simulink model "prMotor"  (R2021a)
settings: Solver=ode3  StartTime=0.0  StopTime=2  FixedStep=0.000125  RelTol=1e-3  EnableMultiTasking=on
values from neighbouring files (symbols this model uses):
  DELTA_EMF = 14    [prMotor_init.m]
  DELTA_THETA = 29    [prMotor_init.m]
  DT_GAIN = 102    [prMotor_init.m]
  DT_IREF_LIM = 205    [prMotor_init.m]
  DT_SET_H = 10    [prMotor_init.m]
  DT_SET_L = -10    [prMotor_init.m]
  DT_VALUE = 2    [prMotor_init.m]
  DUTY = 2048    [prMotor_init.m]
  DUTY_50 = 1024    [prMotor_init.m]
  EMF_GAIN = 759    [prMotor_init.m]
  ID_GAIN = 350    [prMotor_init.m]
  ID_LIM = 205    [prMotor_init.m]
  ID_RPM = 1800    [prMotor_init.m]
  IREF_FLT_A1 = -446    [prMotor_init.m]
  IREF_FLT_B0 = 289    [prMotor_init.m]
  IREF_FLT_B1 = 289    [prMotor_init.m]
  Ki = 0.048828125    [prMotor_init.m]
  mp_emf = [0	3	5	8	10	13	15	18	21	23	26	28	31	33	36	39	41	44	46	49	51	54	56	59	62	64	67	69	72	74	77	79	82	84	87	89	92	94	97	99	102	104	107	109	112	114	117	119	122	124	127	129	132	134	136	139	141	144	146	149	151	153	156	158	161	163	165	168	170	172	175	177	179	182	184	186	189	191	193	195	198	200	202	204	207	209	211	213	216	218	220	222	224	227	229	231	233	235	237	239	242	244	246	248	250	252	254	256	258	260	262 ...(+4035 chars)    [prMotor_init.m]
  mp_sin = [0	6	13	19	25	31	38	44	50	57	63	69	75	82	88	94	100	107	113	119	125	132	138	144	150	156	163	169	175	181	187	194	200	206	212	218	224	230	237	243	249	255	261	267	273	279	285	291	297	303	309	315	321	327	333	339	345	351	357	363	369	374	380	386	392	398	403	409	415	421	426	432	438	443	449	455	460	466	472	477	483	488	494	499	505	510	516	521	526	532	537	543	548	553	558	564	569	574	579	584	590	595	600	605	6 ...(+4281 chars)    [prMotor_init.m]
  mp_theta = [0	1	2	3	4	5	6	7	8	9	10	11	12	13	14	15	16	17	18	19	20	21	22	23	24	25	26	27	28	29	30	31	32	33	34	35	36	37	38	39	40	41	42	43	44	45	46	47	48	49	50	51	52	53	54	55	56	57	58	59	60	61	62	63	64	65	66	67	68	69	70	71	72	73	74	75	76	77	78	79	80	81	82	83	84	85	86	87	88	89	90	91	92	93	94	95	96	97	98	99	100	101	102	103	104	105	106	107	108	109	110	111	112	113	114	115	116	117	118	119	120	121	122	123	124	125	126	1 ...(+3610 chars)    [prMotor_init.m]
  PI_A1 = -1024    [prMotor_init.m]
  PI_B0 = 292    [prMotor_init.m]
  PI_B1 = -279    [prMotor_init.m]
  RPM_GAIN = 15000    [prMotor_init.m]
  RPM_LIM = 3000    [prMotor_init.m]
  RPM_LPF_A1 = -984    [prMotor_init.m]
  RPM_LPF_B0 = 20    [prMotor_init.m]
  RPM_LPF_B1 = 20    [prMotor_init.m]
  T_smp = 0.000125    [prMotor_init.m]
  THETA_ADV_LIM = 85    [prMotor_init.m]
libraries: simulink x1
(part 1 of 2)
settings Model: ModifiedByFormat=GAIO  Creator=GAIO  LastModifiedBy=GAIO
settings SolverCC: AlgebraicLoopSolver=TrustRegion
settings DataIOCC: LimitDataPoints=on  SaveFormat=Array  SignalLoggingSaveFormat=ModelDataLogs  SaveOutput=off  SaveTime=off  ReturnWorkspaceOutputs=off
settings OptimizationCC: ExpressionDepthLimit=2147483647  LifeSpan=1  EfficientTunableParamExpr=on
settings DebuggingCC: UnderspecifiedInitializationDetection=Classic  MergeDetectMultiDrivingBlocksExec=none  SolverPrmCheckMsg=warning  MultiTaskDSMMsg=warning  MultiTaskCondExecSysMsg=none  FcnCallInpInsideContextMsg=warning  StateNameClashWarn=warning  SFUnexpectedBacktrackingDiag=warning  SFNoUnconditionalDefaultTransitionDiag=warning  SFExecutionAtInitializationDiag=none  SFMachineParentedDataDiag=warning  ArithmeticOperatorsInVariantConditions=warning
settings HardwareCC: ProdBitPerPointer=32  ProdBitPerSizeT=32  ProdBitPerPtrDiffT=32  ProdLargestAtomicFloat=None  ProdIntDivRoundTo=Undefined  ProdEndianess=Unspecified  ProdWordSize=32  ProdHWDeviceType=32-bit Generic
settings ModelReferenceCC: PropagateSignalLabelsOutOfModel=off
settings SFSimCC: SimUseLocalCustomCode=off  MATLABDynamicMemAlloc=off  CustomCodeUndefinedFunction=UseInterfaceOnly
settings RTWCC: SystemTargetFile=ert.tlc  TemplateMakefile=ert_default_tmf  RTWUseLocalCustomCode=off
settings CodeAppCC: IgnoreCustomStorageClasses=off  StateflowObjectComments=on
settings ERTTargetCC: MultiwordLength=2048  GenerateSampleERTMain=on  SupportContinuousTime=on  ERTCustomFileTemplate=example_file_process.tlc  ConvertIfToSwitch=off  SuppressUnreachableDefaultCases=off
settings ConfigComp: CovMetricSettings=dcmtrzoibsw  CovSaveCumulativeToWorkspaceVar=on  CovSaveSingleToWorkspaceVar=on  CovSFcnEnable=off  DVMaxProcessTime=7200  DVTestSuiteOptimization=CombinedObjectives (Nonlinear Extended)  DVDetectOutOfBounds=on  DVSaveReport=on

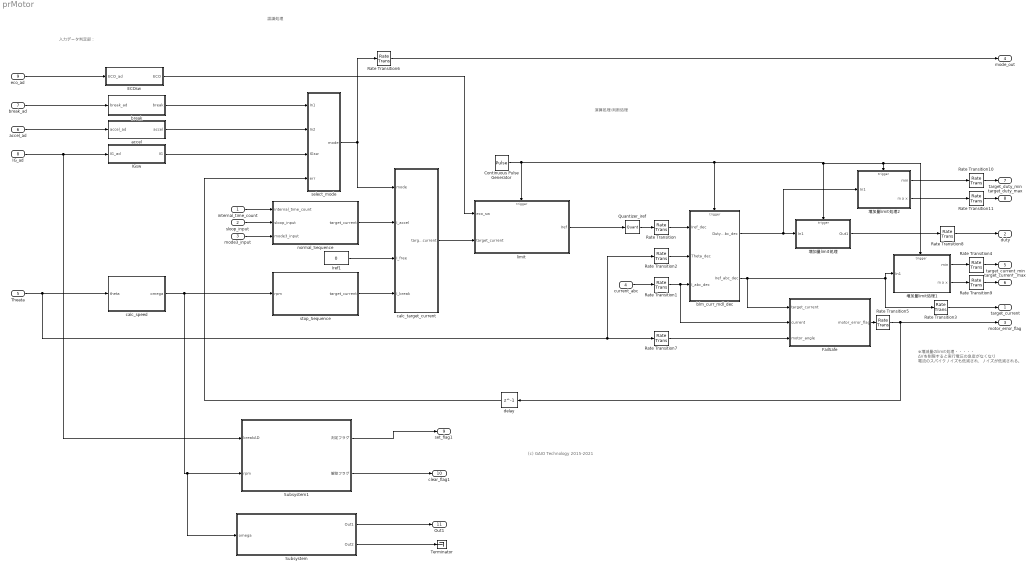
== system prMotor ==
  note: (c) GAIO Technology 2015-2021
  note: 認識処理
  note: 演算処理/判断処理
  note: 入力データ判定部：
  note: ※増減量のlimit処理・・・・・
      | ΔVを制限すると実行電圧の急変がなくなり
      | 電流のスパイクノイズも低減され、ノイズが低減される。
  internal_time_count : Inport  OutDataTypeStr=double  PortDimensions=1  SampleTime=[0.000125,0]
  sloop_input : Inport  Port=2  OutDataTypeStr=double  PortDimensions=1  SampleTime=[0.000125,0]
  mode3_input : Inport  Port=3  OutDataTypeStr=double  PortDimensions=1  SampleTime=[0.000125,0]
  current_abc : Inport  Port=4  OutDataTypeStr=double  PortDimensions=3  SampleTime=[0.000125,0]
  Theata : Inport  Port=5  OutDataTypeStr=double  PortDimensions=1  SampleTime=[0.000125,0]
  accel_ad : Inport  Port=6  SampleTime=[0.000125,0]
  break_ad : Inport  Port=7  SampleTime=[0.000125,0]
  IG_ad : Inport  Port=8  SampleTime=[0.000125,0]
  eco_ad : Inport  Port=9  SampleTime=[0.000125,0]
  Continuous Pulse Generator : DiscretePulseGenerator  PulseType=Time based  Period=T_smp*2  PulseWidth=50
  ECOsw : Subsystem
  FailSafe : Subsystem
  IGsw : Subsystem
  Iref1 : Constant  Value=0
  Quantizer_iref : Quantizer  QuantizationInterval=1
  Rate Transition{,1..4,6..11} (11 alike) : RateTransition
  Rate Transition5 : RateTransition  OutPortSampleTimeOpt=Inherit
  Subsystem : Subsystem
  Subsystem1 : Subsystem
  Terminator : Terminator
  accel : Subsystem
  blm_curr_mdl_dec : Subsystem
  break : Subsystem
  calc_speed : Subsystem
  calc_target_current : Subsystem
  delay : Delay  DelayLength=1  InitialCondition=0
  limit : Subsystem  TreatAsAtomicUnit=on
  normal_Sequence : Subsystem
  select_mode : Subsystem
  stop_Sequence : Subsystem
  増加量limit処理 : Subsystem
  増加量limit処理1 : Subsystem
  増加量limit処理2 : Subsystem
  target_current : Outport  OutDataTypeStr=double  PortDimensions=3  SampleTime=[0.000125,0]
  duty : Outport  Port=2  OutDataTypeStr=double  PortDimensions=3  SampleTime=[0.000125,0]
  motor_error_flag : Outport  Port=3  OutDataTypeStr=boolean  PortDimensions=1  SampleTime=[0.000125,0]
  mode_out : Outport  Port=4  OutDataTypeStr=double  PortDimensions=1  SampleTime=[0.000125,0]
  target_current_min : Outport  Port=5  OutDataTypeStr=double  PortDimensions=3  SampleTime=[0.000125,0]
  target_current＿max : Outport  Port=6  OutDataTypeStr=double  PortDimensions=3  SampleTime=[0.000125,0]
  target_duty_min : Outport  Port=7  OutDataTypeStr=double  PortDimensions=3  SampleTime=[0.000125,0]
  target_duty_max : Outport  Port=8  OutDataTypeStr=double  PortDimensions=3  SampleTime=[0.000125,0]
  set_flag1 : Outport  Port=9  OutDataTypeStr=boolean  PortDimensions=1  SampleTime=[0.000125,0]
  clear_flag1 : Outport  Port=10  OutDataTypeStr=boolean  PortDimensions=1  SampleTime=[0.000125,0]
  Out1 : Outport  Port=11
  wires:
  Rate Transition2/1 -> blm_curr_mdl_dec/2(Theta_dec)
  Rate Transition1/1 -> FailSafe/2(current), blm_curr_mdl_dec/3(I_abc_dec)
  Continuous Pulse Generator/1 -> 増加量limit処理2/Trigger, 増加量limit処理1/Trigger, 増加量limit処理/Trigger, blm_curr_mdl_dec/Trigger, limit/Trigger
  Rate Transition/1 -> blm_curr_mdl_dec/1(Iref_dec)
  current_abc/1 -> Rate Transition1/1
  Quantizer_iref/1 -> Rate Transition/1
  blm_curr_mdl_dec/2(Iref_abc_dec) -> Rate Transition3/1, 増加量limit処理1/1(In1), FailSafe/1(target_current)
  blm_curr_mdl_dec/1(Duty_abc_dec) -> 増加量limit処理2/1(In1), 増加量limit処理/1(In1)
  limit/1(Iref) -> Quantizer_iref/1
  FailSafe/1(motor_error_flag) -> Rate Transition5/1
  Rate Transition5/1 -> motor_error_flag/1, delay/1
  accel_ad/1 -> accel/1(accel_ad)
  break_ad/1 -> break/1(break_ad)
  Rate Transition6/1 -> mode_out/1
  break/1(break) -> select_mode/1(In1)
  accel/1(accel) -> select_mode/2(In2)
  select_mode/1(mode) -> Rate Transition6/1, calc_target_current/1(mode)
  internal_time_count/1 -> normal_Sequence/1(internal_time_count)
  mode3_input/1 -> normal_Sequence/3(mode3_input)
  sloop_input/1 -> normal_Sequence/2(sloop_input)
  normal_Sequence/1(target_current) -> calc_target_current/2(I_accel)
  Iref1/1 -> calc_target_current/3(I_free)
  stop_Sequence/1(target_current) -> calc_target_current/4(I_break)
  Theata/1 -> Rate Transition7/1, Rate Transition2/1, calc_speed/1(theta)
  calc_speed/1(omega) -> Subsystem/1(omega), Subsystem1/2(rpm), stop_Sequence/1(rpm)
  IG_ad/1 -> Subsystem1/1(breakAD), IGsw/1(IG_ad)
  IGsw/1(IG) -> select_mode/3(IGsw)
  Rate Transition7/1 -> FailSafe/3(motor_angle)
  calc_target_current/1(target_current) -> limit/2(target_current)
  eco_ad/1 -> ECOsw/1(ECO_ad)
  ECOsw/1(ECO) -> limit/1(eco_sw)
  delay/1 -> select_mode/4(err)
  増加量limit処理/1(Out1) -> Rate Transition8/1
  増加量limit処理1/1(min) -> Rate Transition4/1
  増加量limit処理1/2(ｍａｘ) -> Rate Transition9/1
  Rate Transition8/1 -> duty/1
  Rate Transition3/1 -> target_current/1
  Rate Transition4/1 -> target_current_min/1
  Rate Transition9/1 -> target_current＿max/1
  Rate Transition11/1 -> target_duty_max/1
  Rate Transition10/1 -> target_duty_min/1
  増加量limit処理2/2(ｍａｘ) -> Rate Transition11/1
  増加量limit処理2/1(min) -> Rate Transition10/1
  Subsystem1/1(判定フラグ) -> set_flag1/1
  Subsystem1/2("解除フラグ　") -> clear_flag1/1
  Subsystem/1(Out1) -> Out1/1
  Subsystem/2(Out2) -> Terminator/1

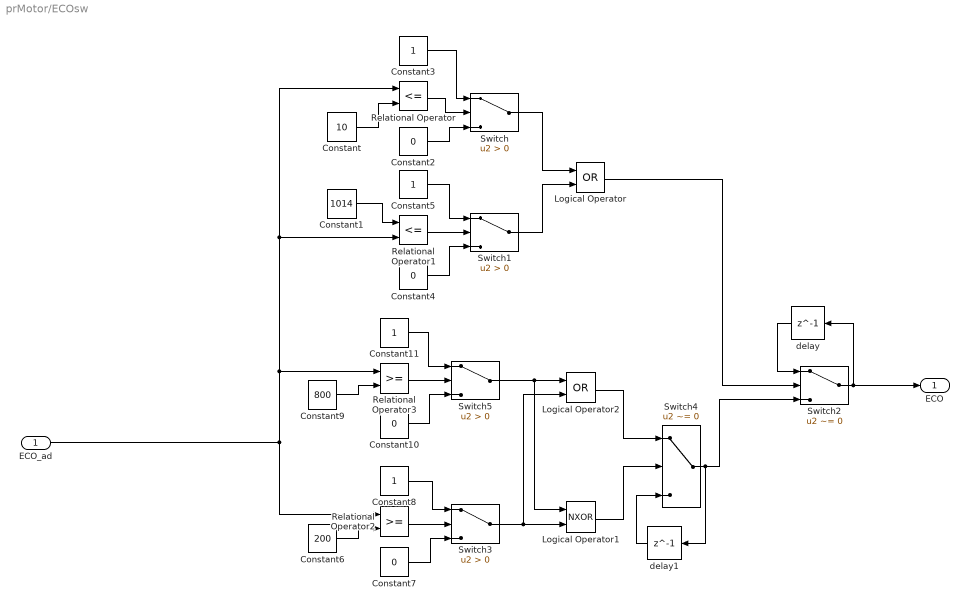
== system prMotor/ECOsw ==
  ECO_ad : Inport
  Constant : Constant  Value=10
  Constant1 : Constant  Value=1014
  Constant{2,4,7,10} (4 alike) : Constant  Value=0
  Constant{3,5,8,11} (4 alike) : Constant
  Constant6 : Constant  Value=200
  Constant9 : Constant  Value=800
  Logical Operator : Logic  Operator=OR  AllPortsSameDT=off  OutDataTypeStr=boolean
  Logical Operator1 : Logic  Operator=NXOR  AllPortsSameDT=off  OutDataTypeStr=boolean
  Logical Operator2 : Logic  Operator=OR  AllPortsSameDT=off  OutDataTypeStr=boolean
  Relational Operator : RelationalOperator  Operator=<=  OutDataTypeStr=boolean  RndMeth=Nearest
  Relational Operator1 : RelationalOperator  Operator=<=  OutDataTypeStr=boolean  RndMeth=Nearest
  Relational Operator2 : RelationalOperator  OutDataTypeStr=boolean  RndMeth=Nearest
  Relational Operator3 : RelationalOperator  OutDataTypeStr=boolean  RndMeth=Nearest
  Switch{,1,3,5} (4 alike) : Switch  Criteria=u2 > Threshold
  Switch2 : Switch  Criteria=u2 ~= 0
  Switch4 : Switch  Criteria=u2 ~= 0
  delay : Delay  DelayLength=1  InitialCondition=0
  delay1 : Delay  DelayLength=1  InitialCondition=0
  ECO : Outport
  wires:
  Logical Operator2/1 -> Switch4/1
  Logical Operator1/1 -> Switch4/2
  ECO_ad/1 -> Relational Operator2/1, Relational Operator3/1, Relational Operator/1, Relational Operator1/2
  Constant10/1 -> Switch5/3
  Constant11/1 -> Switch5/1
  Constant9/1 -> Relational Operator3/2
  Relational Operator3/1 -> Switch5/2
  Switch4/1 -> Switch2/3, delay1/1
  Switch5/1 -> Logical Operator1/1, Logical Operator2/1
  Switch3/1 -> Logical Operator2/2, Logical Operator1/2
  Relational Operator2/1 -> Switch3/2
  Constant6/1 -> Relational Operator2/2
  Constant8/1 -> Switch3/1
  Constant7/1 -> Switch3/3
  Constant2/1 -> Switch/3
  Switch1/1 -> Logical Operator/2
  Constant1/1 -> Relational Operator1/1
  Switch2/1 -> ECO/1, delay/1
  Constant5/1 -> Switch1/1
  Constant3/1 -> Switch/1
  Switch/1 -> Logical Operator/1
  Logical Operator/1 -> Switch2/2
  Constant4/1 -> Switch1/3
  Constant/1 -> Relational Operator/2
  Relational Operator1/1 -> Switch1/2
  Relational Operator/1 -> Switch/2
  delay/1 -> Switch2/1
  delay1/1 -> Switch4/3

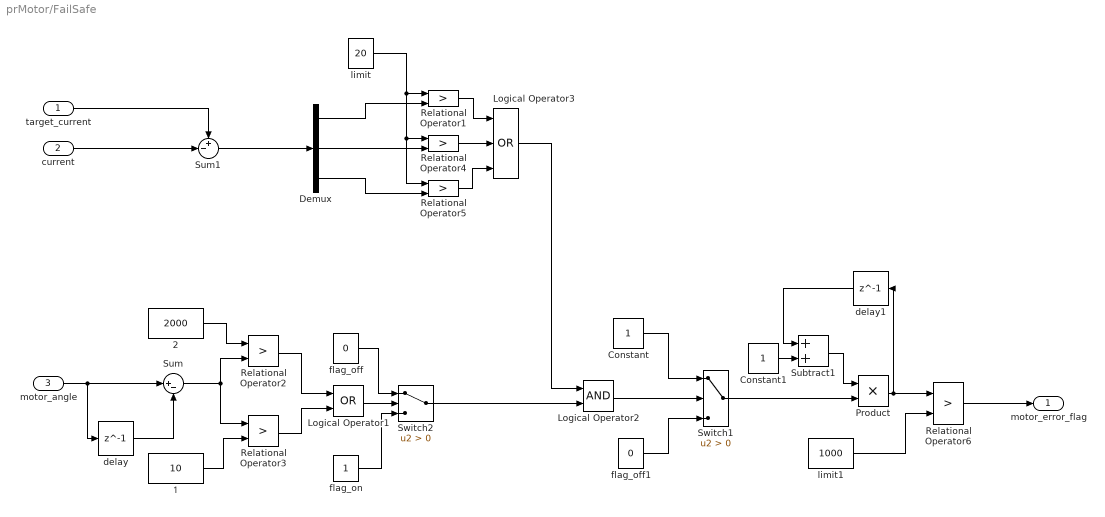
== system prMotor/FailSafe ==
  target_current : Inport  PortDimensions=3
  current : Inport  Port=2  PortDimensions=3
  motor_angle : Inport  Port=3
  2 : Constant  Value=2000
  Constant : Constant
  Constant1 : Constant
  Demux : Demux  Outputs=3
  Logical Operator1 : Logic  Operator=OR  AllPortsSameDT=off  OutDataTypeStr=boolean
  Logical Operator2 : Logic  AllPortsSameDT=off  OutDataTypeStr=boolean
  Logical Operator3 : Logic  Operator=OR  Inputs=3  AllPortsSameDT=off  OutDataTypeStr=boolean
  Product : Product
  Relational Operator{1..6} (6 alike) : RelationalOperator  Operator=>  OutDataTypeStr=boolean  RndMeth=Nearest
  Subtract1 : Sum  InputSameDT=on
  Sum : Sum  Inputs=|+-
  Sum1 : Sum  Inputs=+-|
  Switch1 : Switch  Criteria=u2 > Threshold
  Switch2 : Switch  Criteria=u2 > Threshold
  delay : Delay  DelayLength=1  InitialCondition=0
  delay1 : Delay  DelayLength=1  InitialCondition=0
  flag_off : Constant  Value=0
  flag_off1 : Constant  Value=0
  flag_on : Constant
  limit : Constant  Value=20
  limit1 : Constant  Value=1000
  １ : Constant  Value=10
  motor_error_flag : Outport  OutDataTypeStr=boolean  PortDimensions=1  SampleTime=[0.000125,0]
  wires:
  motor_angle/1 -> Sum/1, delay/1
  2/1 -> Relational Operator2/1
  flag_off/1 -> Switch2/1
  flag_on/1 -> Switch2/3
  Relational Operator2/1 -> Logical Operator1/1
  Logical Operator3/1 -> Logical Operator2/1
  Sum/1 -> Relational Operator3/1, Relational Operator2/2
  limit1/1 -> Relational Operator6/2
  Relational Operator3/1 -> Logical Operator1/2
  Sum1/1 -> Demux/1
  Relational Operator5/1 -> Logical Operator3/3
  Switch2/1 -> Logical Operator2/2
  flag_off1/1 -> Switch1/3
  Relational Operator4/1 -> Logical Operator3/2
  Logical Operator1/1 -> Switch2/2
  limit/1 -> Relational Operator5/1, Relational Operator4/1, Relational Operator1/1
  １/1 -> Relational Operator3/2
  Constant/1 -> Switch1/1
  Relational Operator1/1 -> Logical Operator3/1
  target_current/1 -> Sum1/1
  current/1 -> Sum1/2
  Relational Operator6/1 -> motor_error_flag/1
  Logical Operator2/1 -> Switch1/2
  Constant1/1 -> Subtract1/2
  Switch1/1 -> Product/2
  Product/1 -> Relational Operator6/1, delay1/1
  Subtract1/1 -> Product/1
  Demux/1 -> Relational Operator1/2
  Demux/2 -> Relational Operator4/2
  Demux/3 -> Relational Operator5/2
  delay/1 -> Sum/2
  delay1/1 -> Subtract1/1

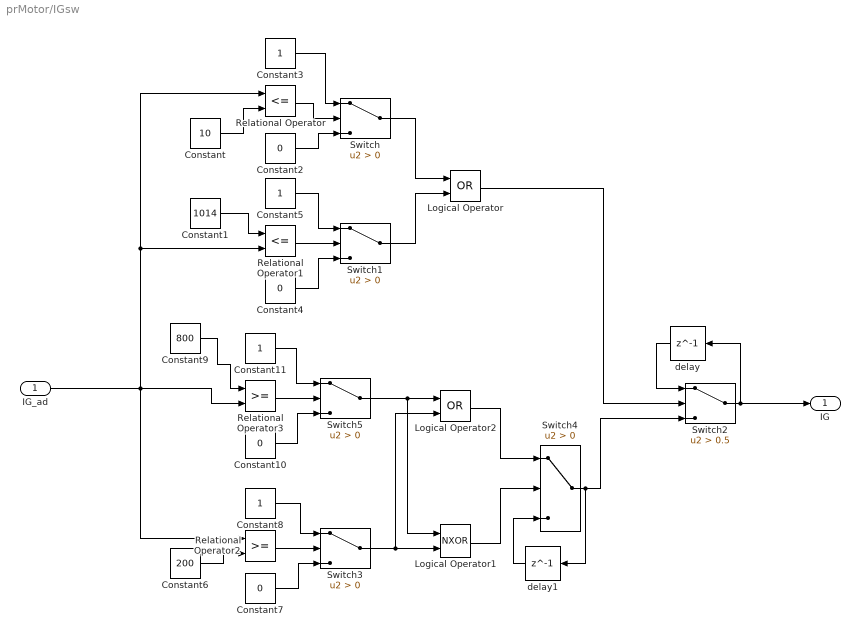
== system prMotor/IGsw ==
  IG_ad : Inport
  Constant : Constant  Value=10
  Constant1 : Constant  Value=1014
  Constant{2,4,7,10} (4 alike) : Constant  Value=0
  Constant{3,5,8,11} (4 alike) : Constant
  Constant6 : Constant  Value=200
  Constant9 : Constant  Value=800
  Logical Operator : Logic  Operator=OR  AllPortsSameDT=off  OutDataTypeStr=boolean
  Logical Operator1 : Logic  Operator=NXOR  AllPortsSameDT=off  OutDataTypeStr=boolean
  Logical Operator2 : Logic  Operator=OR  AllPortsSameDT=off  OutDataTypeStr=boolean
  Relational Operator : RelationalOperator  Operator=<=  OutDataTypeStr=boolean  RndMeth=Nearest
  Relational Operator1 : RelationalOperator  Operator=<=  OutDataTypeStr=boolean  RndMeth=Nearest
  Relational Operator2 : RelationalOperator  OutDataTypeStr=boolean  RndMeth=Nearest
  Relational Operator3 : RelationalOperator  OutDataTypeStr=boolean  RndMeth=Nearest
  Switch{,1,3..5} (5 alike) : Switch  Criteria=u2 > Threshold
  Switch2 : Switch  Criteria=u2 > Threshold  Threshold=0.5
  delay : Delay  DelayLength=1  InitialCondition=0
  delay1 : Delay  DelayLength=1  InitialCondition=0
  IG : Outport
  wires:
  Relational Operator/1 -> Switch/2
  Relational Operator1/1 -> Switch1/2
  Constant/1 -> Relational Operator/2
  Constant4/1 -> Switch1/3
  Logical Operator/1 -> Switch2/2
  Switch/1 -> Logical Operator/1
  Constant3/1 -> Switch/1
  Constant5/1 -> Switch1/1
  Switch2/1 -> IG/1, delay/1
  Constant1/1 -> Relational Operator1/1
  Switch1/1 -> Logical Operator/2
  Constant2/1 -> Switch/3
  Constant7/1 -> Switch3/3
  Constant8/1 -> Switch3/1
  Constant6/1 -> Relational Operator2/2
  Relational Operator2/1 -> Switch3/2
  Switch3/1 -> Logical Operator1/2, Logical Operator2/2
  Switch5/1 -> Logical Operator2/1, Logical Operator1/1
  Switch4/1 -> Switch2/3, delay1/1
  Relational Operator3/1 -> Switch5/2
  Constant9/1 -> Relational Operator3/1
  Constant11/1 -> Switch5/1
  Constant10/1 -> Switch5/3
  IG_ad/1 -> Relational Operator3/2, Relational Operator2/1, Relational Operator1/2, Relational Operator/1
  Logical Operator1/1 -> Switch4/2
  Logical Operator2/1 -> Switch4/1
  delay/1 -> Switch2/1
  delay1/1 -> Switch4/3

== system prMotor/Subsystem ==
  omega : Inport
  Abs1 : Abs
  Add : Sum
  Add1 : Sum  Inputs=+-
  Constant : Constant
  Constant1 : Constant  Value=2
  Data Type Conversion : DataTypeConversion  OutDataTypeStr=boolean  RndMeth=Round
  Data Type Conversion1 : DataTypeConversion  OutDataTypeStr=boolean  RndMeth=Zero
  Logical Operator2 : Logic  Operator=OR  OutDataTypeStr=boolean
  Logical Operator3 : Logic  Operator=XOR  AllPortsSameDT=off  OutDataTypeStr=boolean
  Product : Product
  Saturation : Saturate  UpperLimit=10  LowerLimit=2
  Sign1 : Signum
  Sign2 : Signum
  Out1 : Outport
  Out2 : Outport  Port=2
  wires:
  Logical Operator2/1 -> Out1/1  "３"
  omega/1 -> Sign1/1, Abs1/1
  Product/1 -> Saturation/1
  Add/1 -> Data Type Conversion/1, Product/1
  Logical Operator3/1 -> Out2/1  "４"
  Add1/1 -> Sign2/1
  Saturation/1 -> Add1/1
  Constant/1 -> Add/2
  Constant1/1 -> Add1/2
  Abs1/1 -> Product/2
  Data Type Conversion/1 -> Logical Operator3/1, Logical Operator2/1  "1"
  Data Type Conversion1/1 -> Logical Operator2/2, Logical Operator3/2  "2"
  Sign2/1 -> Data Type Conversion1/1
  Sign1/1 -> Add/1

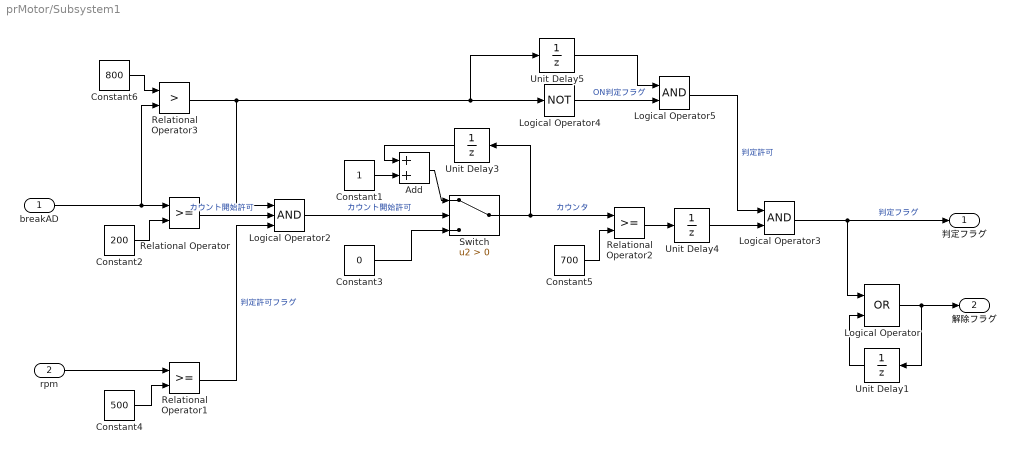
== system prMotor/Subsystem1 ==
  breakAD : Inport
  rpm : Inport  Port=2
  Add : Sum
  Constant1 : Constant
  Constant2 : Constant  Value=200
  Constant3 : Constant  Value=0
  Constant4 : Constant  Value=500
  Constant5 : Constant  Value=700
  Constant6 : Constant  Value=800
  Logical Operator : Logic  Operator=OR  AllPortsSameDT=off  OutDataTypeStr=boolean
  Logical Operator2 : Logic  Inputs=3  AllPortsSameDT=off  OutDataTypeStr=boolean
  Logical Operator3 : Logic  AllPortsSameDT=off  OutDataTypeStr=boolean
  Logical Operator4 : Logic  Operator=NOT  AllPortsSameDT=off  OutDataTypeStr=boolean
  Logical Operator5 : Logic  AllPortsSameDT=off  OutDataTypeStr=boolean
  Relational Operator : RelationalOperator  OutDataTypeStr=boolean  RndMeth=Simplest
  Relational Operator1 : RelationalOperator  OutDataTypeStr=boolean  RndMeth=Simplest
  Relational Operator2 : RelationalOperator  OutDataTypeStr=boolean  RndMeth=Simplest
  Relational Operator3 : RelationalOperator  Operator=>  OutDataTypeStr=boolean  RndMeth=Simplest
  Switch : Switch  Criteria=u2 > Threshold
  Unit Delay{1,3..5} (4 alike) : UnitDelay  SampleTime=-1  HasFrameUpgradeWarning=on
  判定フラグ : Outport  VectorParamsAs1DForOutWhenUnconnected=off
  "解除フラグ　" : Outport  Port=2  VectorParamsAs1DForOutWhenUnconnected=off
  wires:
  Relational Operator/1 -> Logical Operator2/2  "カウント開始許可"
  Logical Operator5/1 -> Logical Operator3/1  "判定許可"
  Constant1/1 -> Add/2
  Logical Operator2/1 -> Switch/2  "カウント開始許可"
  Switch/1 -> Unit Delay3/1, Relational Operator2/1  "カウンタ"
  Logical Operator/1 -> "解除フラグ　"/1, Unit Delay1/1
  Unit Delay5/1 -> Logical Operator5/1
  Relational Operator2/1 -> Unit Delay4/1
  Logical Operator4/1 -> Logical Operator5/2  "ON判定フラグ"
  Add/1 -> Switch/1
  Unit Delay3/1 -> Add/1
  breakAD/1 -> Relational Operator/1, Relational Operator3/2
  Unit Delay4/1 -> Logical Operator3/2
  Relational Operator1/1 -> Logical Operator2/3  "判定許可フラグ"
  Constant6/1 -> Relational Operator3/1
  Relational Operator3/1 -> Logical Operator2/1, Unit Delay5/1, Logical Operator4/1
  Constant4/1 -> Relational Operator1/2
  Constant5/1 -> Relational Operator2/2
  Unit Delay1/1 -> Logical Operator/2
  Logical Operator3/1 -> 判定フラグ/1, Logical Operator/1  "判定フラグ"
  Constant2/1 -> Relational Operator/2
  Constant3/1 -> Switch/3
  rpm/1 -> Relational Operator1/1

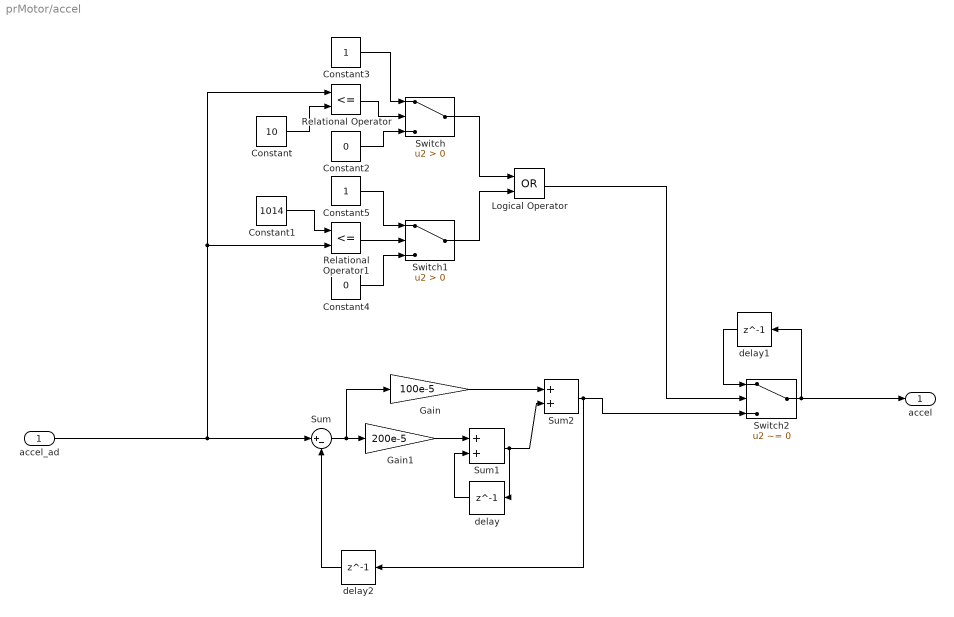
== system prMotor/accel ==
  accel_ad : Inport
  Constant : Constant  Value=10
  Constant1 : Constant  Value=1014
  Constant2 : Constant  Value=0
  Constant3 : Constant
  Constant4 : Constant  Value=0
  Constant5 : Constant
  Gain : Gain  Gain=100e-5
  Gain1 : Gain  Gain=200e-5
  Logical Operator : Logic  Operator=OR  AllPortsSameDT=off  OutDataTypeStr=boolean
  Relational Operator : RelationalOperator  Operator=<=  OutDataTypeStr=boolean  RndMeth=Nearest
  Relational Operator1 : RelationalOperator  Operator=<=  OutDataTypeStr=boolean  RndMeth=Nearest
  Sum : Sum  Inputs=|+-
  Sum1 : Sum
  Sum2 : Sum
  Switch : Switch  Criteria=u2 > Threshold
  Switch1 : Switch  Criteria=u2 > Threshold
  Switch2 : Switch  Criteria=u2 ~= 0
  delay : Delay  DelayLength=1  InitialCondition=0
  delay1 : Delay  DelayLength=1  InitialCondition=0
  delay2 : Delay  DelayLength=1  InitialCondition=0
  accel : Outport
  wires:
  accel_ad/1 -> Sum/1, Relational Operator/1, Relational Operator1/2
  Sum1/1 -> Sum2/2, delay/1
  Constant2/1 -> Switch/3
  Sum2/1 -> Switch2/3, delay2/1
  Switch1/1 -> Logical Operator/2
  Constant1/1 -> Relational Operator1/1
  Switch2/1 -> accel/1, delay1/1
  Constant5/1 -> Switch1/1
  Constant3/1 -> Switch/1
  Switch/1 -> Logical Operator/1
  Logical Operator/1 -> Switch2/2
  Gain/1 -> Sum2/1
  Constant4/1 -> Switch1/3
  Constant/1 -> Relational Operator/2
  Relational Operator1/1 -> Switch1/2
  Relational Operator/1 -> Switch/2
  Gain1/1 -> Sum1/1
  Sum/1 -> Gain1/1, Gain/1
  delay/1 -> Sum1/2
  delay1/1 -> Switch2/1
  delay2/1 -> Sum/2

== system prMotor/blm_curr_mdl_dec ==
  Iref_dec : Inport
  Theta_dec : Inport  Port=2
  I_abc_dec : Inport  Port=3
  Trigger : TriggerPort  VariantControl=(inherit)  PortDimensions=1
  DT_comp_dec : Subsystem
  Duty_calc_dec : Subsystem
  Emf_comp_dec : Subsystem
  FB_calc_dec : Subsystem
  Iref_calc_dec : Subsystem
  Rpm_calc_dec : Subsystem
  Theta_calc_dec : Subsystem
  Vector_calc_dec : Subsystem
  Duty_abc_dec : Outport
  Iref_abc_dec : Outport  Port=2
  wires:
  Iref_dec/1 -> DT_comp_dec/1(Iref), Iref_calc_dec/1(Iref)
  Emf_comp_dec/1(EMF_abc) -> Duty_calc_dec/3(EMF_abc)
  DT_comp_dec/1(DT_abc) -> Duty_calc_dec/1(DT_abc)
  FB_calc_dec/1(PI_abc) -> Duty_calc_dec/2(PI_abc)
  Duty_calc_dec/1(Duty_abc) -> Duty_abc_dec/1
  Theta_calc_dec/1(Theta_adv) -> Vector_calc_dec/3(Theta)
  Vector_calc_dec/1(Iref_abc) -> FB_calc_dec/1(Iref_abc), Iref_abc_dec/1, DT_comp_dec/2(Iref_abc)
  I_abc_dec/1 -> FB_calc_dec/2(I_abc)
  Rpm_calc_dec/1(Rpm) -> Emf_comp_dec/2(Rpm), Theta_calc_dec/2(Rpm), Iref_calc_dec/2(Rpm)
  Theta_dec/1 -> Rpm_calc_dec/1(Theta), Theta_calc_dec/1(Theta), Emf_comp_dec/1(Theta)
  Iref_calc_dec/2(Id) -> Vector_calc_dec/2(Id)
  Iref_calc_dec/1(Iq) -> Vector_calc_dec/1(Iq)

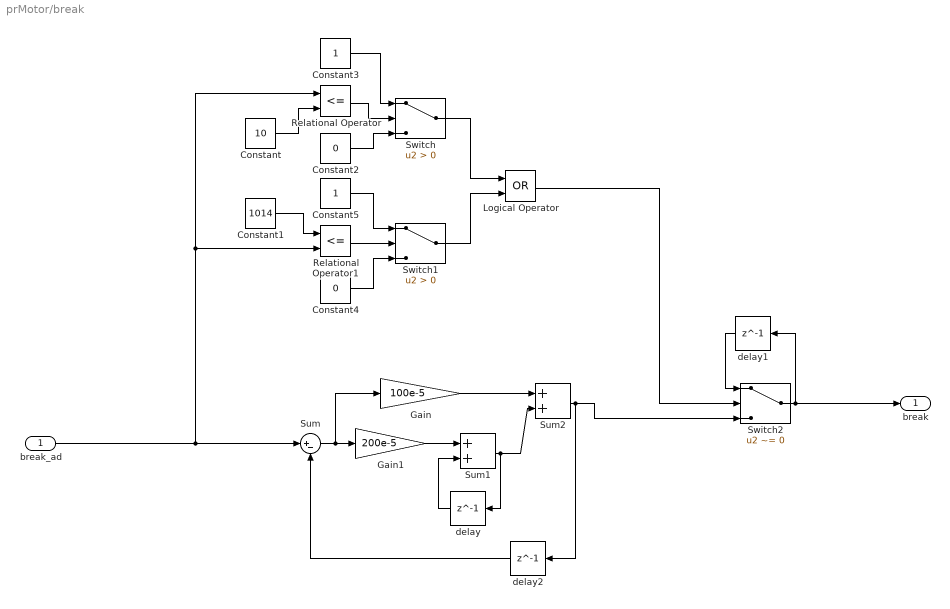
== system prMotor/break ==
  break_ad : Inport
  Constant : Constant  Value=10
  Constant1 : Constant  Value=1014
  Constant2 : Constant  Value=0
  Constant3 : Constant
  Constant4 : Constant  Value=0
  Constant5 : Constant
  Gain : Gain  Gain=100e-5
  Gain1 : Gain  Gain=200e-5
  Logical Operator : Logic  Operator=OR  AllPortsSameDT=off  OutDataTypeStr=boolean
  Relational Operator : RelationalOperator  Operator=<=  OutDataTypeStr=boolean  RndMeth=Nearest
  Relational Operator1 : RelationalOperator  Operator=<=  OutDataTypeStr=boolean  RndMeth=Nearest
  Sum : Sum  Inputs=|+-
  Sum1 : Sum
  Sum2 : Sum
  Switch : Switch  Criteria=u2 > Threshold
  Switch1 : Switch  Criteria=u2 > Threshold
  Switch2 : Switch  Criteria=u2 ~= 0
  delay : Delay  DelayLength=1  InitialCondition=0
  delay1 : Delay  DelayLength=1  InitialCondition=0
  delay2 : Delay  DelayLength=1  InitialCondition=0
  break : Outport
  wires:
  Sum/1 -> Gain/1, Gain1/1
  Gain1/1 -> Sum1/1
  Relational Operator/1 -> Switch/2
  Relational Operator1/1 -> Switch1/2
  Constant/1 -> Relational Operator/2
  Constant4/1 -> Switch1/3
  Gain/1 -> Sum2/1
  Logical Operator/1 -> Switch2/2
  Switch/1 -> Logical Operator/1
  Constant3/1 -> Switch/1
  Constant5/1 -> Switch1/1
  Switch2/1 -> break/1, delay1/1
  Constant1/1 -> Relational Operator1/1
  Switch1/1 -> Logical Operator/2
  Sum2/1 -> Switch2/3, delay2/1
  Constant2/1 -> Switch/3
  Sum1/1 -> Sum2/2, delay/1
  break_ad/1 -> Relational Operator1/2, Relational Operator/1, Sum/1
  delay/1 -> Sum1/2
  delay1/1 -> Switch2/1
  delay2/1 -> Sum/2

== system prMotor/calc_speed ==
  theta : Inport
  Sum : Sum  Inputs=|+-
  delay : Delay  DelayLength=1  InitialCondition=0
  omega : Outport
  wires:
  Sum/1 -> omega/1
  theta/1 -> Sum/1, delay/1
  delay/1 -> Sum/2

== system prMotor/calc_target_current ==
  mode : Inport
  I_accel : Inport  Port=2
  I_free : Inport  Port=3
  I_break : Inport  Port=4
  Multiport Switch : MultiPortSwitch  DiagnosticForDefault=None
  target_current : Outport
  wires:
  I_break/1 -> Multiport Switch/4
  I_accel/1 -> Multiport Switch/2
  I_free/1 -> Multiport Switch/3
  mode/1 -> Multiport Switch/1
  Multiport Switch/1 -> target_current/1

== system prMotor/limit ==
  eco_sw : Inport
  target_current : Inport  Port=2
  Trigger : TriggerPort  VariantControl=(inherit)  PortDimensions=1
  Constant1 : Constant  Value=5
  Constant2 : Constant  Value=20
  Divide : Product  Inputs=/*
  Divide1 : Product  Inputs=/*
  Gain : Gain  Gain=-1
  Sum : Sum  Inputs=+-|
  Sum1 : Sum  Inputs=++|
  Sum2 : Sum  Inputs=|++
  Switch1 : Switch  Threshold=1
  Switch2 : Switch  Criteria=u2 > Threshold
  Switch3 : Switch  Threshold=1
  Switch4 : Switch  Threshold=1
  delay : Delay  DelayLength=1  InitialCondition=0
  Iref : Outport
  wires:
  eco_sw/1 -> Switch1/2
  Sum2/1 -> Switch3/1
  Divide/1 -> Switch4/2
  Divide1/1 -> Switch3/2
  Switch2/1 -> Iref/1, delay/1
  Switch3/1 -> Switch2/3
  Switch1/1 -> Divide/1, Sum1/1, Gain/1
  Sum/1 -> Switch2/2, Divide1/2, Divide/2
  Constant2/1 -> Switch1/3
  target_current/1 -> Switch4/3, Sum/1, Switch3/3
  Sum1/1 -> Switch4/1
  Switch4/1 -> Switch2/1
  Constant1/1 -> Switch1/1
  Gain/1 -> Sum2/2, Divide1/1
  delay/1 -> Sum1/2, Sum/2, Sum2/1

== system prMotor/normal_Sequence ==
  internal_time_count : Inport
  sloop_input : Inport  Port=2
  mode3_input : Inport  Port=3
  Iref : Constant  Value=200
  Iref1 : Constant  Value=300
  Iref_dec : Gain  Gain=1/Ki
  Logical Operator : Logic  AllPortsSameDT=off  OutDataTypeStr=boolean
  Multiport Switch : MultiPortSwitch  DiagnosticForDefault=None
  Product1 : Product  RndMeth=Zero
  Product2 : Product  RndMeth=Zero
  Relational Operator : RelationalOperator  Operator=>  OutDataTypeStr=boolean  RndMeth=Nearest
  Relational Operator1 : RelationalOperator  Operator=>  OutDataTypeStr=boolean  RndMeth=Nearest
  Switch : Switch  Criteria=u2 > Threshold
  Switch1 : Switch  Criteria=u2 > Threshold
  input_mode : Constant
  input_mode1 : Constant  Value=2
  input_mode2 : Constant  Value=3
  target_current : Outport
  wires:
  mode3_input/1 -> Product2/1
  sloop_input/1 -> Product1/1
  Switch1/1 -> Multiport Switch/1
  Logical Operator/1 -> Switch1/2
  Relational Operator1/1 -> Logical Operator/1
  Product2/1 -> Multiport Switch/3
  input_mode2/1 -> Switch1/1
  Relational Operator/1 -> Logical Operator/2, Switch/2
  input_mode1/1 -> Switch/1
  Iref1/1 -> Relational Operator1/1
  Product1/1 -> Multiport Switch/2
  input_mode/1 -> Switch/3
  Iref/1 -> Relational Operator/2, Iref_dec/1
  internal_time_count/1 -> Relational Operator/1, Relational Operator1/2
  Multiport Switch/1 -> target_current/1
  Switch/1 -> Switch1/3
  Iref_dec/1 -> Multiport Switch/4, Product1/2, Product2/2

== system prMotor/select_mode ==
  In1 : Inport
  In2 : Inport  Port=2
  IGsw : Inport  Port=3
  err : Inport  Port=4  OutDataTypeStr=boolean
  Logical Operator : Logic  Operator=OR  AllPortsSameDT=off  OutDataTypeStr=boolean
  Logical Operator1 : Logic  Operator=NOT  AllPortsSameDT=off  OutDataTypeStr=boolean
  Relational Operator : RelationalOperator  Operator=>  OutDataTypeStr=boolean  RndMeth=Nearest
  Relational Operator1 : RelationalOperator  Operator=>  OutDataTypeStr=boolean  RndMeth=Nearest
  Switch1 : Switch  Criteria=u2 > Threshold
  Switch2 : Switch  Criteria=u2 > Threshold
  Switch3 : Switch  Criteria=u2 > Threshold
  accel_off : Constant  Value=150
  break_on : Constant  Value=10
  mode1 : Constant
  mode2 : Constant  Value=2
  mode2_1 : Constant  Value=2
  mode3 : Constant  Value=3
  mode : Outport
  wires:
  In1/1 -> Relational Operator/1
  mode3/1 -> Switch1/1
  Relational Operator/1 -> Switch1/2
  accel_off/1 -> Relational Operator1/1
  Relational Operator1/1 -> Switch2/2
  mode1/1 -> Switch2/3
  mode2/1 -> Switch2/1
  break_on/1 -> Relational Operator/2
  Switch2/1 -> Switch1/3
  In2/1 -> Relational Operator1/2
  Switch1/1 -> Switch3/3
  IGsw/1 -> Logical Operator1/1
  err/1 -> Logical Operator/2
  Logical Operator/1 -> Switch3/2
  mode2_1/1 -> Switch3/1
  Switch3/1 -> mode/1
  Logical Operator1/1 -> Logical Operator/1

== system prMotor/stop_Sequence ==
  rpm : Inport
  Logical Operator1 : Logic  AllPortsSameDT=off  OutDataTypeStr=boolean
  Multiport Switch1 : MultiPortSwitch  DiagnosticForDefault=None
  Product : Product  Inputs=**/
  Relational Operator2 : RelationalOperator  Operator=>  OutDataTypeStr=boolean  RndMeth=Nearest
  Relational Operator3 : RelationalOperator  Operator=>  OutDataTypeStr=boolean  RndMeth=Nearest
  Saturation Dynamic : simulink/Discontinuities/Saturation Dynamic  OutMin=[]  OutMax=[]  OutDataTypeStr=Inherit: Same as second input  OutDataType=fixdt(1, 16)  OutScaling=2^-10  DoSatur=off
  Sum : Sum  Inputs=-+|
  Sum1 : Sum  Inputs=+-|
  Switch2 : Switch  Criteria=u2 > Threshold
  Switch3 : Switch  Criteria=u2 > Threshold
  break_mode4 : Constant  Value=-160
  break_mode5 : Constant  Value=-10
  input_mode3 : Constant
  input_mode4 : Constant  Value=3
  input_mode5 : Constant  Value=2
  max_spd : Constant  Value=160
  min_spd : Constant  Value=10
  target_current : Outport
  wires:
  Sum/1 -> Product/1
  Product/1 -> Multiport Switch1/3
  input_mode5/1 -> Switch3/1
  input_mode4/1 -> Switch2/1
  Logical Operator1/1 -> Switch3/2
  Multiport Switch1/1 -> target_current/1
  Switch2/1 -> Switch3/3
  break_mode5/1 -> Multiport Switch1/4, Product/2
  input_mode3/1 -> Switch2/3
  max_spd/1 -> Relational Operator3/1, Sum1/1, Saturation Dynamic/1
  min_spd/1 -> Sum1/2, Saturation Dynamic/3, Relational Operator2/2, Sum/1
  rpm/1 -> Relational Operator3/2, Relational Operator2/1, Saturation Dynamic/2
  Relational Operator3/1 -> Logical Operator1/1
  break_mode4/1 -> Multiport Switch1/2
  Relational Operator2/1 -> Switch2/2, Logical Operator1/2
  Switch3/1 -> Multiport Switch1/1
  Saturation Dynamic/1 -> Sum/2
  Sum1/1 -> Product/3

== system prMotor/増加量limit処理 ==
  In1 : Inport
  Trigger : TriggerPort  VariantControl=Variant  PortDimensions=1
  Constant4 : Constant  Value=5
  Constant5 : Constant  Value=-5
  Sum : Sum  Inputs=+-|
  Sum1 : Sum  Inputs=++|
  Sum2 : Sum  Inputs=|++
  Switch2 : Switch  Criteria=u2 > Threshold
  Switch3 : Switch  Criteria=u2 > Threshold  Threshold=-5
  Switch4 : Switch  Criteria=u2 > Threshold  Threshold=5
  Unit Delay : UnitDelay  SampleTime=-1  HasFrameUpgradeWarning=on
  Out1 : Outport
  wires:
  Sum/1 -> Switch3/2, Switch2/2, Switch4/2
  Unit Delay/1 -> Sum1/2, Sum2/1, Sum/2
  Sum2/1 -> Switch3/3
  Constant4/1 -> Sum1/1
  In1/1 -> Switch3/1, Sum/1, Switch4/3
  Switch3/1 -> Switch2/3
  Switch4/1 -> Switch2/1
  Sum1/1 -> Switch4/1
  Constant5/1 -> Sum2/2
  Switch2/1 -> Unit Delay/1, Out1/1

== system prMotor/増加量limit処理1 ==
  In1 : Inport
  Trigger : TriggerPort  VariantControl=Variant  PortDimensions=1
  Constant1 : Constant  Value=-1000
  Constant2 : Constant  Value=1000
  Constant4 : Constant  Value=5
  Constant5 : Constant  Value=-5
  MinMax : MinMax  Inputs=2
  MinMax1 : MinMax  Function=max  Inputs=2
  Sum : Sum  Inputs=+-|
  Sum1 : Sum  Inputs=++|
  Sum2 : Sum  Inputs=|++
  Switch2 : Switch  Criteria=u2 > Threshold
  Switch3 : Switch  Criteria=u2 > Threshold  Threshold=-5
  Switch4 : Switch  Criteria=u2 > Threshold  Threshold=5
  Unit Delay : UnitDelay  SampleTime=-1  HasFrameUpgradeWarning=on
  min : Outport
  ｍａｘ : Outport  Port=2
  wires:
  Constant5/1 -> Sum2/2
  Sum1/1 -> Switch4/1
  Switch4/1 -> Switch2/1
  Switch3/1 -> Switch2/3
  In1/1 -> Switch4/3, Sum/1, Switch3/1
  Constant4/1 -> Sum1/1
  Sum2/1 -> Switch3/3
  Unit Delay/1 -> Sum2/1, Sum/2, Sum1/2
  Sum/1 -> Switch4/2, Switch2/2, Switch3/2
  Constant1/1 -> MinMax/2
  MinMax/1 -> min/1
  MinMax1/1 -> ｍａｘ/1
  Constant2/1 -> MinMax1/2
  Switch2/1 -> Unit Delay/1, MinMax1/1, MinMax/1

== system prMotor/増加量limit処理2 ==
  In1 : Inport
  Trigger : TriggerPort  VariantControl=Variant  PortDimensions=1
  Constant1 : Constant  Value=-1000
  Constant2 : Constant  Value=1000
  Constant4 : Constant  Value=5
  Constant5 : Constant  Value=-5
  MinMax : MinMax  Inputs=2
  MinMax1 : MinMax  Function=max  Inputs=2
  Sum : Sum  Inputs=+-|
  Sum1 : Sum  Inputs=++|
  Sum2 : Sum  Inputs=|++
  Switch2 : Switch  Criteria=u2 > Threshold
  Switch3 : Switch  Criteria=u2 > Threshold  Threshold=-5
  Switch4 : Switch  Criteria=u2 > Threshold  Threshold=5
  Unit Delay : UnitDelay  SampleTime=-1  HasFrameUpgradeWarning=on
  min : Outport
  ｍａｘ : Outport  Port=2
  wires:
  Switch2/1 -> Unit Delay/1, MinMax/1, MinMax1/1
  Constant2/1 -> MinMax1/2
  MinMax1/1 -> ｍａｘ/1
  MinMax/1 -> min/1
  Constant1/1 -> MinMax/2
  Sum/1 -> Switch3/2, Switch2/2, Switch4/2
  Unit Delay/1 -> Sum1/2, Sum/2, Sum2/1
  Sum2/1 -> Switch3/3
  Constant4/1 -> Sum1/1
  In1/1 -> Switch3/1, Sum/1, Switch4/3
  Switch3/1 -> Switch2/3
  Switch4/1 -> Switch2/1
  Sum1/1 -> Switch4/1
  Constant5/1 -> Sum2/2

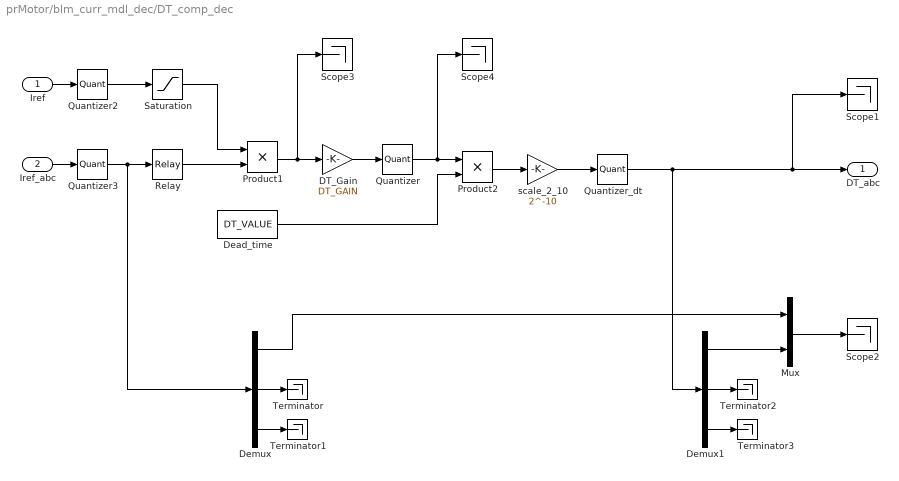
== system prMotor/blm_curr_mdl_dec/DT_comp_dec ==
  Iref : Inport
  Iref_abc : Inport  Port=2
  DT_Gain : Gain  Gain=DT_GAIN
  Dead_time : Constant  Value=DT_VALUE
  Demux : Demux  Outputs=3
  Demux1 : Demux  Outputs=3
  Mux : Mux  Inputs=2
  Product1 : Product  RndMeth=Zero
  Product2 : Product  RndMeth=Zero
  Quantizer : Quantizer  QuantizationInterval=1
  Quantizer2 : Quantizer  QuantizationInterval=1
  Quantizer3 : Quantizer  QuantizationInterval=1
  Quantizer_dt : Quantizer  QuantizationInterval=1
  Relay : Relay  OnSwitchValue=DT_SET_H  OffSwitchValue=DT_SET_L  OffOutputValue=-1
  Saturation : Saturate  UpperLimit=DT_IREF_LIM  LowerLimit=-DT_IREF_LIM
  Scope{1..4} (4 alike) : Terminator
  Terminator{,1..3} (4 alike) : Terminator
  scale_2_10 : Gain  Gain=2^-10
  DT_abc : Outport
  wires:
  Quantizer3/1 -> Demux/1, Relay/1
  Quantizer2/1 -> Saturation/1
  Quantizer_dt/1 -> Demux1/1, Scope1/1, DT_abc/1
  Quantizer/1 -> Scope4/1, Product2/1
  scale_2_10/1 -> Quantizer_dt/1
  DT_Gain/1 -> Quantizer/1
  Dead_time/1 -> Product2/2
  Mux/1 -> Scope2/1
  Demux1/1 -> Mux/2
  Demux/1 -> Mux/1
  Demux1/3 -> Terminator3/1
  Demux1/2 -> Terminator2/1
  Demux/3 -> Terminator1/1
  Demux/2 -> Terminator/1
  Saturation/1 -> Product1/1
  Product2/1 -> scale_2_10/1
  Product1/1 -> DT_Gain/1, Scope3/1
  Relay/1 -> Product1/2
  Iref_abc/1 -> Quantizer3/1
  Iref/1 -> Quantizer2/1

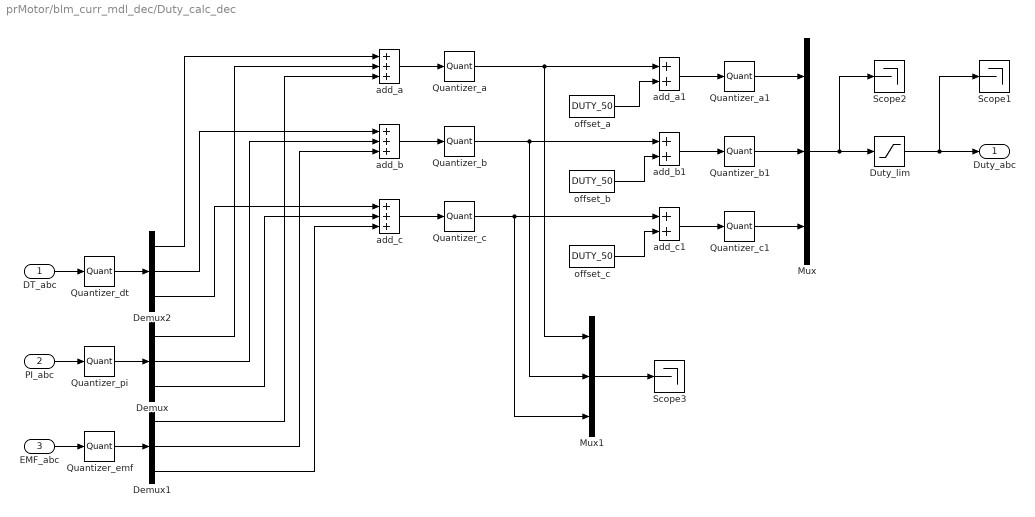
== system prMotor/blm_curr_mdl_dec/Duty_calc_dec ==
  DT_abc : Inport
  PI_abc : Inport  Port=2
  EMF_abc : Inport  Port=3
  Demux : Demux  Outputs=3
  Demux1 : Demux  Outputs=3
  Demux2 : Demux  Outputs=3
  Duty_lim : Saturate  UpperLimit=DUTY-1  LowerLimit=0
  Mux : Mux  Inputs=3
  Mux1 : Mux  Inputs=3
  Quantizer_a : Quantizer  QuantizationInterval=1
  Quantizer_a1 : Quantizer  QuantizationInterval=1
  Quantizer_b : Quantizer  QuantizationInterval=1
  Quantizer_b1 : Quantizer  QuantizationInterval=1
  Quantizer_c : Quantizer  QuantizationInterval=1
  Quantizer_c1 : Quantizer  QuantizationInterval=1
  Quantizer_dt : Quantizer  QuantizationInterval=1
  Quantizer_emf : Quantizer  QuantizationInterval=1
  Quantizer_pi : Quantizer  QuantizationInterval=1
  Scope1 : Terminator
  Scope2 : Terminator
  Scope3 : Terminator
  add_a : Sum  Inputs=+++
  add_a1 : Sum
  add_b : Sum  Inputs=+++
  add_b1 : Sum
  add_c : Sum  Inputs=+++
  add_c1 : Sum
  offset_a : Constant  Value=DUTY_50
  offset_b : Constant  Value=DUTY_50
  offset_c : Constant  Value=DUTY_50
  Duty_abc : Outport
  wires:
  Quantizer_emf/1 -> Demux1/1
  Quantizer_pi/1 -> Demux/1
  Quantizer_dt/1 -> Demux2/1
  Mux1/1 -> Scope3/1
  Quantizer_c/1 -> Mux1/3, add_c1/1
  Quantizer_b/1 -> Mux1/2, add_b1/1
  Quantizer_a/1 -> Mux1/1, add_a1/1
  Quantizer_c1/1 -> Mux/3
  Quantizer_b1/1 -> Mux/2
  Quantizer_a1/1 -> Mux/1
  Duty_lim/1 -> Scope1/1, Duty_abc/1
  add_b/1 -> Quantizer_b/1
  Demux1/3 -> add_c/3
  Demux1/2 -> add_b/3
  Demux/3 -> add_c/2
  Demux1/1 -> add_a/3
  Demux/2 -> add_b/2
  Demux/1 -> add_a/2
  Demux2/3 -> add_c/1
  Demux2/2 -> add_b/1
  Demux2/1 -> add_a/1
  add_c/1 -> Quantizer_c/1
  add_a/1 -> Quantizer_a/1
  offset_c/1 -> add_c1/2
  add_c1/1 -> Quantizer_c1/1
  add_b1/1 -> Quantizer_b1/1
  offset_b/1 -> add_b1/2
  offset_a/1 -> add_a1/2
  add_a1/1 -> Quantizer_a1/1
  EMF_abc/1 -> Quantizer_emf/1
  DT_abc/1 -> Quantizer_dt/1
  PI_abc/1 -> Quantizer_pi/1
  Mux/1 -> Scope2/1, Duty_lim/1

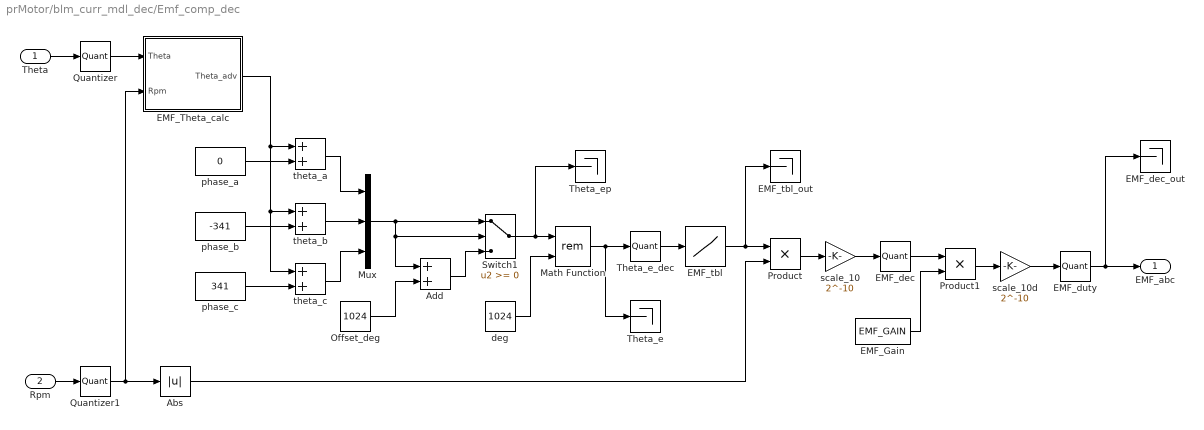
== system prMotor/blm_curr_mdl_dec/Emf_comp_dec ==
  Theta : Inport
  Rpm : Inport  Port=2
  Abs : Abs
  Add : Sum
  EMF_Gain : Constant  Value=EMF_GAIN
  EMF_Theta_calc : Subsystem
  EMF_dec : Quantizer  QuantizationInterval=1
  EMF_dec_out : Terminator
  EMF_duty : Quantizer  QuantizationInterval=1
  EMF_tbl : Lookup  InputValues=mp_theta  Table=mp_emf  RndMeth=Round  SaturateOnIntegerOverflow=on
  EMF_tbl_out : Terminator
  Math Function : Math  Operator=rem  SignedPower=on  SaturateOnIntegerOverflow=on
  Mux : Mux  Inputs=3
  Offset_deg : Constant  Value=1024
  Product : Product  RndMeth=Zero
  Product1 : Product  RndMeth=Zero
  Quantizer : Quantizer  QuantizationInterval=1
  Quantizer1 : Quantizer  QuantizationInterval=1
  Switch1 : Switch
  Theta_e : Terminator
  Theta_e_dec : Quantizer  QuantizationInterval=1
  Theta_ep : Terminator
  deg : Constant  Value=1024
  phase_a : Constant  Value=0
  phase_b : Constant  Value=-341
  phase_c : Constant  Value=341
  scale_10 : Gain  Gain=2^-10
  scale_10d : Gain  Gain=2^-10
  theta_a : Sum
  theta_b : Sum
  theta_c : Sum
  EMF_abc : Outport
  wires:
  EMF_Gain/1 -> Product1/2
  EMF_duty/1 -> EMF_dec_out/1, EMF_abc/1
  Product1/1 -> scale_10d/1
  scale_10d/1 -> EMF_duty/1
  EMF_dec/1 -> Product1/1
  Quantizer1/1 -> Abs/1, EMF_Theta_calc/2(Rpm)
  EMF_Theta_calc/1(Theta_adv) -> theta_b/1, theta_c/1, theta_a/1
  Quantizer/1 -> EMF_Theta_calc/1(Theta)
  scale_10/1 -> EMF_dec/1
  Theta_e_dec/1 -> EMF_tbl/1
  EMF_tbl/1 -> Product/1, EMF_tbl_out/1
  Abs/1 -> Product/2
  Math Function/1 -> Theta_e/1, Theta_e_dec/1
  Switch1/1 -> Theta_ep/1, Math Function/1
  Mux/1 -> Switch1/2, Add/1, Switch1/1
  Offset_deg/1 -> Add/2
  Add/1 -> Switch1/3
  deg/1 -> Math Function/2
  Theta/1 -> Quantizer/1
  phase_a/1 -> theta_a/2
  theta_a/1 -> Mux/1
  theta_c/1 -> Mux/3
  theta_b/1 -> Mux/2
  phase_c/1 -> theta_c/2
  phase_b/1 -> theta_b/2
  Product/1 -> scale_10/1
  Rpm/1 -> Quantizer1/1

== system prMotor/blm_curr_mdl_dec/FB_calc_dec ==
  Iref_abc : Inport
  I_abc : Inport  Port=2
  PI_calc_dec : Subsystem
  Quantizer_iabc : Quantizer  QuantizationInterval=1
  Quantizer_iref_abc : Quantizer  QuantizationInterval=1
  sub : Sum  Inputs=+-
  PI_abc : Outport
  wires:
  Quantizer_iabc/1 -> sub/2
  Quantizer_iref_abc/1 -> sub/1
  PI_calc_dec/1(Out) -> PI_abc/1
  sub/1 -> PI_calc_dec/1(In)
  I_abc/1 -> Quantizer_iabc/1
  Iref_abc/1 -> Quantizer_iref_abc/1

== system prMotor/blm_curr_mdl_dec/Iref_calc_dec ==
  Iref : Inport
  Rpm : Inport  Port=2
  Dead Zone : DeadZone  LowerValue=-ID_RPM  UpperValue=ID_RPM  SaturateOnIntegerOverflow=on
  Id_Gain : Constant  Value=ID_GAIN
  Id_lim : Saturate  UpperLimit=ID_LIM  LowerLimit=-ID_LIM
  Iref_flt : Subsystem
  Iref_lim : Saturate  UpperLimit=2048  LowerLimit=-2048
  Mux : Mux  Inputs=2
  Mux1 : Mux  Inputs=2
  Product : Product  RndMeth=Zero
  Quantizer : Quantizer  QuantizationInterval=1
  Quantizer_iref : Quantizer  QuantizationInterval=1
  Quantizer_rpm : Quantizer  QuantizationInterval=1
  Scope1 : Terminator
  Scope2 : Terminator
  scale : Gain  Gain=2^-10
  Iq : Outport
  Id : Outport  Port=2
  wires:
  Quantizer_rpm/1 -> Dead Zone/1
  Quantizer_iref/1 -> Iref_lim/1
  Iref_lim/1 -> Iref_flt/1(In), Mux/1
  Quantizer/1 -> Mux1/1, Id_lim/1
  Mux1/1 -> Scope2/1
  Id_Gain/1 -> Product/2
  Product/1 -> scale/1
  Dead Zone/1 -> Product/1
  scale/1 -> Quantizer/1
  Id_lim/1 -> Mux1/2, Id/1
  Mux/1 -> Scope1/1
  Rpm/1 -> Quantizer_rpm/1
  Iref_flt/1(Out) -> Mux/2, Iq/1
  Iref/1 -> Quantizer_iref/1

== system prMotor/blm_curr_mdl_dec/Rpm_calc_dec ==
  Theta : Inport
  Add : Sum
  Product : Product  RndMeth=Zero
  Quantizer : Quantizer  QuantizationInterval=1
  Quantizer1 : Quantizer  QuantizationInterval=1
  Rpm_Gain : Constant  Value=RPM_GAIN
  Rpm_lpf : Subsystem
  Subtract : Sum  Inputs=+-
  Subtract2 : Sum  Inputs=+-
  Switch : Switch  Criteria=u2 > Threshold  Threshold=-700
  Switch1 : Switch  Criteria=u2 > Threshold  Threshold=700
  delay : Delay  DelayLength=1  InitialCondition=0
  delay1 : Delay  DelayLength=1  InitialCondition=0
  offset1 : Constant  Value=1024
  offset2 : Constant  Value=1024
  rpm_lim : Saturate  UpperLimit=RPM_LIM  LowerLimit=-RPM_LIM
  scale_2_8 : Gain  Gain=2^-8
  Rpm : Outport
  wires:
  scale_2_8/1 -> Quantizer/1
  Rpm_Gain/1 -> Product/2
  Quantizer1/1 -> Subtract/1, delay/1
  Quantizer/1 -> Rpm_lpf/1(In)
  Product/1 -> scale_2_8/1
  rpm_lim/1 -> Rpm/1
  offset1/1 -> Subtract2/2
  Switch1/1 -> Product/1
  Subtract2/1 -> Switch1/1
  Rpm_lpf/1(Out) -> rpm_lim/1
  Add/1 -> Switch/3
  offset2/1 -> Add/2
  Switch/1 -> Switch1/3
  Subtract/1 -> Subtract2/1, Switch1/2, Switch/1, Switch/2, Add/1
  Theta/1 -> Quantizer1/1
  delay/1 -> delay1/1
  delay1/1 -> Subtract/2

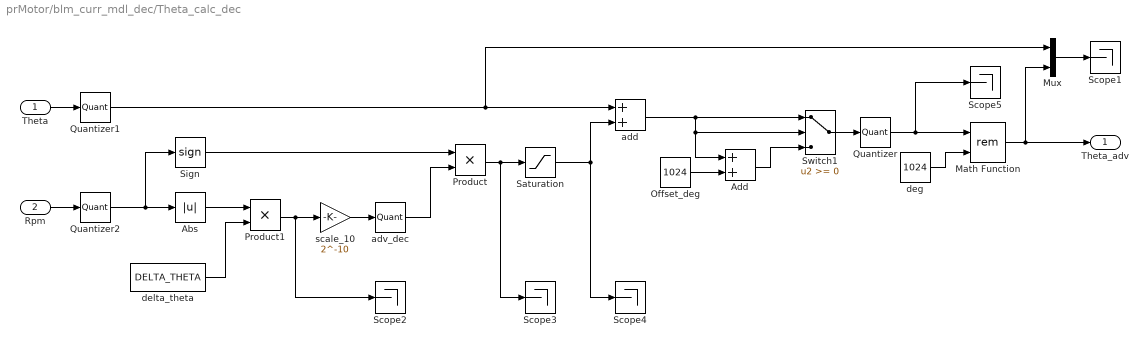
== system prMotor/blm_curr_mdl_dec/Theta_calc_dec ==
  Theta : Inport
  Rpm : Inport  Port=2
  Abs : Abs
  Add : Sum
  Math Function : Math  Operator=rem  SignedPower=on  SaturateOnIntegerOverflow=on
  Mux : Mux  Inputs=2
  Offset_deg : Constant  Value=1024
  Product : Product  RndMeth=Zero
  Product1 : Product  RndMeth=Zero
  Quantizer : Quantizer  QuantizationInterval=1
  Quantizer1 : Quantizer  QuantizationInterval=1
  Quantizer2 : Quantizer  QuantizationInterval=1
  Saturation : Saturate  UpperLimit=THETA_ADV_LIM  LowerLimit=-THETA_ADV_LIM
  Scope{1..5} (5 alike) : Terminator
  Sign : Signum
  Switch1 : Switch
  add : Sum
  adv_dec : Quantizer  QuantizationInterval=1
  deg : Constant  Value=1024
  delta_theta : Constant  Value=DELTA_THETA
  scale_10 : Gain  Gain=2^-10  RndMeth=Round
  Theta_adv : Outport
  wires:
  Saturation/1 -> Scope4/1, add/2
  Quantizer2/1 -> Sign/1, Abs/1
  Quantizer1/1 -> Mux/1, add/1
  Quantizer/1 -> Scope5/1, Math Function/1
  adv_dec/1 -> Product/2
  delta_theta/1 -> Product1/2
  Abs/1 -> Product1/1
  scale_10/1 -> adv_dec/1
  Switch1/1 -> Quantizer/1
  add/1 -> Switch1/2, Add/1, Switch1/1
  Offset_deg/1 -> Add/2
  Add/1 -> Switch1/3
  Math Function/1 -> Mux/2, Theta_adv/1
  deg/1 -> Math Function/2
  Mux/1 -> Scope1/1
  Product/1 -> Scope3/1, Saturation/1
  Product1/1 -> Scope2/1, scale_10/1
  Sign/1 -> Product/1
  Rpm/1 -> Quantizer2/1
  Theta/1 -> Quantizer1/1

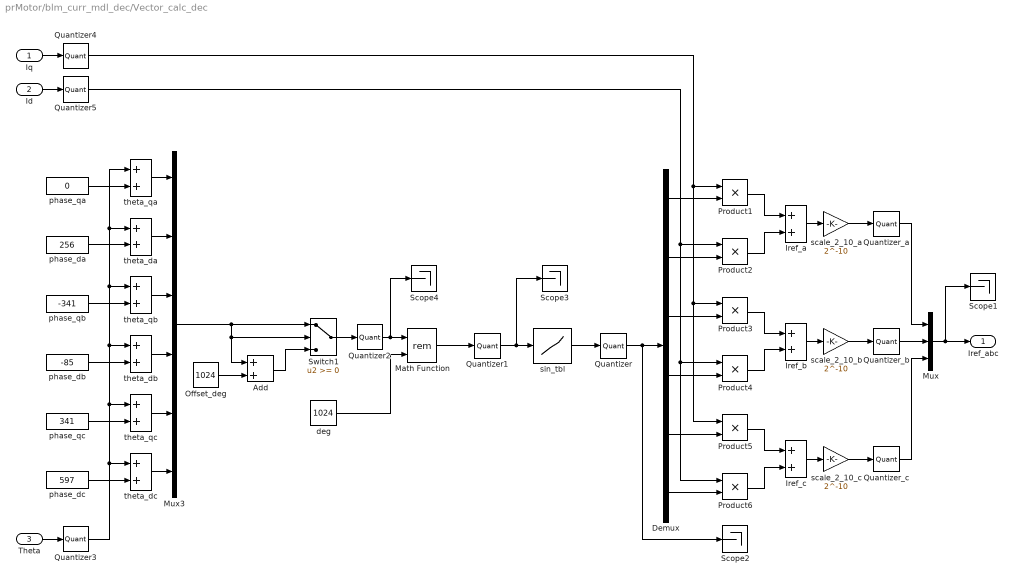
== system prMotor/blm_curr_mdl_dec/Vector_calc_dec ==
  Iq : Inport
  Id : Inport  Port=2
  Theta : Inport  Port=3
  Add : Sum
  Demux : Demux  Outputs=6
  Iref_a : Sum
  Iref_b : Sum
  Iref_c : Sum
  Math Function : Math  Operator=rem  SignedPower=on  SaturateOnIntegerOverflow=on
  Mux : Mux  Inputs=3
  Mux3 : Mux  Inputs=6
  Offset_deg : Constant  Value=1024
  Product{1..6} (6 alike) : Product  RndMeth=Zero
  Quantizer{,1..5} (6 alike) : Quantizer  QuantizationInterval=1
  Quantizer_a : Quantizer  QuantizationInterval=1
  Quantizer_b : Quantizer  QuantizationInterval=1
  Quantizer_c : Quantizer  QuantizationInterval=1
  Scope{1..4} (4 alike) : Terminator
  Switch1 : Switch
  deg : Constant  Value=1024
  phase_da : Constant  Value=256
  phase_db : Constant  Value=-85
  phase_dc : Constant  Value=597
  phase_qa : Constant  Value=0
  phase_qb : Constant  Value=-341
  phase_qc : Constant  Value=341
  scale_2_10_a : Gain  Gain=2^-10
  scale_2_10_b : Gain  Gain=2^-10
  scale_2_10_c : Gain  Gain=2^-10
  sin_tbl : Lookup  InputValues=mp_theta  Table=mp_sin  RndMeth=Round  SaturateOnIntegerOverflow=on
  theta_da : Sum
  theta_db : Sum
  theta_dc : Sum
  theta_qa : Sum
  theta_qb : Sum
  theta_qc : Sum
  Iref_abc : Outport
  wires:
  Quantizer5/1 -> Product6/1, Product4/1, Product2/1
  Quantizer4/1 -> Product5/1, Product3/1, Product1/1
  Quantizer3/1 -> theta_dc/1, theta_da/1, theta_qa/1, theta_qb/1, theta_db/1, theta_qc/1
  Quantizer2/1 -> Scope4/1, Math Function/1
  Quantizer_c/1 -> Mux/3
  Quantizer_b/1 -> Mux/2
  Quantizer_a/1 -> Mux/1
  scale_2_10_c/1 -> Quantizer_c/1
  scale_2_10_b/1 -> Quantizer_b/1
  scale_2_10_a/1 -> Quantizer_a/1
  Quantizer/1 -> Scope2/1, Demux/1
  Quantizer1/1 -> Scope3/1, sin_tbl/1
  Iref_c/1 -> scale_2_10_c/1
  Demux/6 -> Product6/2
  Demux/5 -> Product5/2
  Product6/1 -> Iref_c/2
  Product5/1 -> Iref_c/1
  Demux/4 -> Product4/2
  Demux/3 -> Product3/2
  Iref_b/1 -> scale_2_10_b/1
  Product4/1 -> Iref_b/2
  Product3/1 -> Iref_b/1
  Mux/1 -> Scope1/1, Iref_abc/1
  Iref_a/1 -> scale_2_10_a/1
  Id/1 -> Quantizer5/1
  Demux/2 -> Product2/2
  Product2/1 -> Iref_a/2
  Product1/1 -> Iref_a/1
  Iq/1 -> Quantizer4/1
  Demux/1 -> Product1/2
  sin_tbl/1 -> Quantizer/1
  theta_da/1 -> Mux3/2
  Math Function/1 -> Quantizer1/1
  Switch1/1 -> Quantizer2/1
  Mux3/1 -> Switch1/2, Add/1, Switch1/1
  Offset_deg/1 -> Add/2
  Add/1 -> Switch1/3
  deg/1 -> Math Function/2
  phase_qc/1 -> theta_qc/2
  theta_qc/1 -> Mux3/5
  theta_dc/1 -> Mux3/6
  phase_dc/1 -> theta_dc/2
  phase_qb/1 -> theta_qb/2
  theta_qb/1 -> Mux3/3
  theta_db/1 -> Mux3/4
  phase_db/1 -> theta_db/2
  Theta/1 -> Quantizer3/1
  phase_qa/1 -> theta_qa/2
  theta_qa/1 -> Mux3/1
  phase_da/1 -> theta_da/2

== system prMotor/blm_curr_mdl_dec/Emf_comp_dec/EMF_Theta_calc ==
  Theta : Inport
  Rpm : Inport  Port=2
  Abs : Abs
  Add : Sum
  Math Function : Math  Operator=rem  SignedPower=on  SaturateOnIntegerOverflow=on
  Mux : Mux  Inputs=2
  Offset_deg : Constant  Value=1024
  Product : Product  RndMeth=Zero
  Product1 : Product  RndMeth=Zero
  Scope1 : Terminator
  Scope2 : Terminator
  Scope3 : Terminator
  Sign : Signum
  Switch1 : Switch
  add : Sum
  adv_dec : Quantizer  QuantizationInterval=1
  deg : Constant  Value=1024
  delta_emf : Constant  Value=DELTA_EMF
  scale_10 : Gain  Gain=2^-10
  Theta_adv : Outport
  wires:
  adv_dec/1 -> Product/2
  delta_emf/1 -> Product1/2
  Abs/1 -> Product1/1
  scale_10/1 -> adv_dec/1
  Switch1/1 -> Math Function/1
  add/1 -> Switch1/2, Add/1, Switch1/1
  Offset_deg/1 -> Add/2
  Add/1 -> Switch1/3
  Math Function/1 -> Mux/2, Theta_adv/1
  deg/1 -> Math Function/2
  Mux/1 -> Scope1/1
  Product/1 -> Scope3/1, add/2
  Product1/1 -> Scope2/1, scale_10/1
  Sign/1 -> Product/1
  Rpm/1 -> Sign/1, Abs/1
  Theta/1 -> Mux/1, add/1

== system prMotor/blm_curr_mdl_dec/FB_calc_dec/PI_calc_dec ==
  In : Inport
  Demux : Demux  Outputs=3
  Mux : Mux  Inputs=3
  PI_cont_a : Subsystem
  PI_cont_b : Subsystem
  PI_cont_c : Subsystem
  Out : Outport
  wires:
  PI_cont_c/1(Out) -> Mux/3
  Mux/1 -> Out/1
  PI_cont_b/1(Out) -> Mux/2
  PI_cont_a/1(Out) -> Mux/1
  Demux/3 -> PI_cont_c/1(In)
  Demux/2 -> PI_cont_b/1(In)
  Demux/1 -> PI_cont_a/1(In)
  In/1 -> Demux/1

== system prMotor/blm_curr_mdl_dec/Iref_calc_dec/Iref_flt ==
  In : Inport
  Add : Sum
  IREF_FLT_A1 : Gain  Gain=IREF_FLT_A1
  IREF_FLT_B0 : Gain  Gain=IREF_FLT_B0
  IREF_FLT_B1 : Gain  Gain=IREF_FLT_B1
  Quantizer : Quantizer  QuantizationInterval=1
  Quantizer1 : Quantizer  QuantizationInterval=1
  Quantizer2 : Quantizer  QuantizationInterval=1
  Scale_2_10_a : Gain  Gain=2^-10
  Scale_2_10_b : Gain  Gain=2^-10
  Scope1 : Terminator
  Sub : Sum  Inputs=+-
  delay : Delay  DelayLength=1  InitialCondition=0
  Out : Outport
  wires:
  Quantizer/1 -> Sub/1
  Quantizer1/1 -> Sub/2
  Quantizer2/1 -> Out/1
  Scale_2_10_a/1 -> Quantizer1/1
  Scale_2_10_b/1 -> Quantizer2/1
  IREF_FLT_A1/1 -> Scale_2_10_a/1
  IREF_FLT_B1/1 -> Add/2
  IREF_FLT_B0/1 -> Add/1
  Add/1 -> Scale_2_10_b/1
  Sub/1 -> IREF_FLT_B0/1, delay/1, Scope1/1
  In/1 -> Quantizer/1
  delay/1 -> IREF_FLT_A1/1, IREF_FLT_B1/1

== system prMotor/blm_curr_mdl_dec/Rpm_calc_dec/Rpm_lpf ==
  In : Inport
  Add : Sum
  Quantizer : Quantizer  QuantizationInterval=1
  Quantizer1 : Quantizer  QuantizationInterval=1
  Quantizer2 : Quantizer  QuantizationInterval=1
  RPM_LPF_A1 : Gain  Gain=RPM_LPF_A1
  RPM_LPF_B0 : Gain  Gain=RPM_LPF_B0
  RPM_LPF_B1 : Gain  Gain=RPM_LPF_B1
  Scale_2_10_a : Gain  Gain=2^-10
  Scale_2_10_b : Gain  Gain=2^-10
  Scope1 : Terminator
  Sub : Sum  Inputs=+-
  delay : Delay  DelayLength=1  InitialCondition=0
  Out : Outport
  wires:
  Quantizer/1 -> Sub/1
  Quantizer1/1 -> Sub/2
  Quantizer2/1 -> Out/1
  Scale_2_10_a/1 -> Quantizer1/1
  Scale_2_10_b/1 -> Quantizer2/1
  RPM_LPF_A1/1 -> Scale_2_10_a/1
  RPM_LPF_B1/1 -> Add/2
  RPM_LPF_B0/1 -> Add/1
  Add/1 -> Scale_2_10_b/1
  Sub/1 -> RPM_LPF_B0/1, delay/1, Scope1/1
  In/1 -> Quantizer/1
  delay/1 -> RPM_LPF_A1/1, RPM_LPF_B1/1

== system prMotor/blm_curr_mdl_dec/FB_calc_dec/PI_calc_dec/PI_cont_a ==
  In : Inport
  Add : Sum
  PI_A1 : Gain  Gain=PI_A1
  PI_B0 : Gain  Gain=PI_B0
  PI_B1 : Gain  Gain=PI_B1
  Quantizer : Quantizer  QuantizationInterval=1
  Quantizer1 : Quantizer  QuantizationInterval=1
  Scale_2_10_a : Gain  Gain=2^-10
  Scale_2_10_b : Gain  Gain=2^-10
  Sub : Sum  Inputs=+-
  delay : Delay  DelayLength=1  InitialCondition=T_smp
  Out : Outport
  wires:
  Quantizer1/1 -> Sub/2
  Quantizer/1 -> Out/1
  Scale_2_10_a/1 -> Quantizer1/1
  Scale_2_10_b/1 -> Quantizer/1
  PI_A1/1 -> Scale_2_10_a/1
  PI_B1/1 -> Add/2
  PI_B0/1 -> Add/1
  Add/1 -> Scale_2_10_b/1
  Sub/1 -> PI_B0/1, delay/1
  In/1 -> Sub/1
  delay/1 -> PI_A1/1, PI_B1/1
